simulink model "Counter_mod5"  (R2020a)
settings: Solver=VariableStepAuto  StartTime=0.0  StopTime=10  RelTol=1e-3
undefined symbols (not defined in the file): sigbuilder_block
settings Model: Creator=Shivam  LastModifiedBy=Shivam

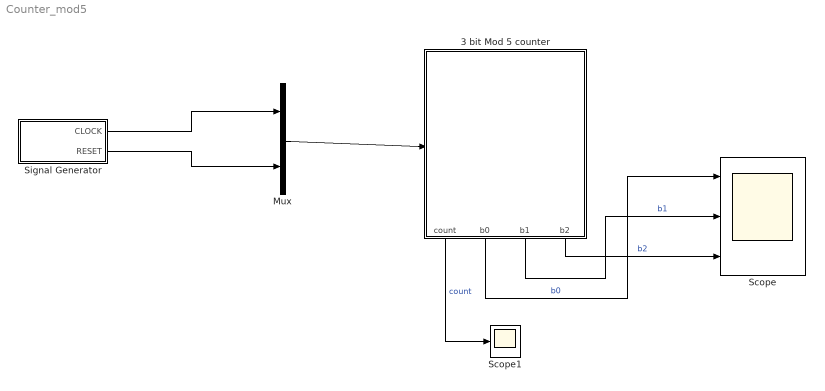
== system Counter_mod5 ==
  3 bit Mod 5 counter : Stateflow chart  TreatAsAtomicUnit=on
  Mux : Mux  Inputs=2
  Scope : Scope  NumInputPorts=3
  Scope1 : Scope
  Signal Generator : Subsystem  Tag=STV Subsys  LoadFcn=sigbuilder_block('load');  StartFcn=sigbuilder_block('start');  StopFcn=sigbuilder_block('stop');  ClipboardFcn=sigbuilder_block('clipboard');  mask(Sigbuilder block){tuvar=[0:10]}
      mask help: Simulink:masks:SigbuilderBlock_MD
      mask init:
      | if ~strcmp(get_param(bdroot(gcbh),'SimulationStatus'),'stopped') tuvar = sigbuilder_block('maskInit'); end
      settings: CopyFcn=sigbuilder_block('copy');  DeleteFcn=sigbuilder_block('delete');  ModelCloseFcn=sigbuilder_block('modelClose');  PreSaveFcn=sigbuilder_block('preSave');  PauseFcn=sigbuilder_block('pause');  ContinueFcn=sigbuilder_block('continue');  NameChangeFcn=sigbuilder_block('namechange');  OpenFcn=sigbuilder_block('open',[283.5 133.5 550.5 359.25 ]);  CloseFcn=sigbuilder_block('close');
      mask Display: plot(0, 0, 100, 100,[2, 2, 32, 32, 2], [68, 8, 8, 68, 68],[32, 2], [38, 38], [32, 19, 2],[53, 60, 44], [32, 17, 17, 2],[16, 16, 31, 31]);txt = getActiveGroup(gcbh);text(2, 100, txt,'verticalAlignment', 'top');
  wires:
  Mux/1 -> 3 bit Mod 5 counter/Trigger
  Signal Generator/1(CLOCK) -> Mux/1
  Signal Generator/2(RESET) -> Mux/2
  3 bit Mod 5 counter/2(b0) -> Scope/1  "b0"
  3 bit Mod 5 counter/3(b1) -> Scope/2  "b1"
  3 bit Mod 5 counter/4(b2) -> Scope/3  "b2"
  3 bit Mod 5 counter/1(count) -> Scope1/1  "count"

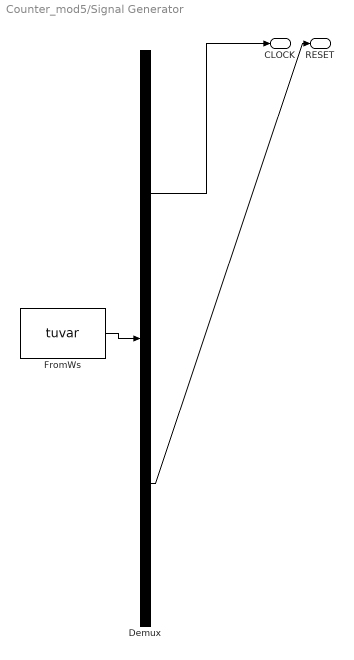
== system Counter_mod5/Signal Generator ==
  Demux : Demux  Tag=STV Demux  Outputs=2
      settings: DisplayOption=none
  FromWs : FromWorkspace  Tag=STV FromWs  VariableName=tuvar
      SigBuilderData=|
      | common.afterFinalStr = 'Extrapolate'
      | common.sampleTime = 0
      | dataSet.timeRange = [0 10]
      | dataSet.name = 'Group 1'
      | sbobj.Groups.Name = 'Group 1'
      | sbobj.Groups.Signals(1).Name = 'CLOCK'
      | sbobj.Groups.Signals(1).XData = [0 0.5 0.5 1 1 1.5 1.5 2 2 2.5 2.5 3 3 3.5 3.5 4 4 4.5 4.5 5 5 5.5 5.5 6 6 6.5 6.5 7 7 7.5 7.5 8 8 8.5 8.5 9 9 9.5 9.5 10]
      | sbobj.Groups.Signals(1).YData = [1 1 0 0 1 1 0 0 1 1 0 0 1 1 0 0 1 1 0 0 1 1 0 0 1 1 0 0 1 1 0 0 1 1 0 0 1 1 0 0]
      | sbobj.Groups.Signals(2).Name = 'RESET'
      | sbobj.Groups.Signals(2).XData = [0 7.98 7.98 9.02 9.02 10]
      | sbobj.Groups.Signals(2).YData = [0 0 1.02 1.02 0 0]
  CLOCK : Outport  Tag=STV Outport
  RESET : Outport  Tag=STV Outport  Port=2
  wires:
  FromWs/1 -> Demux/1
  Demux/1 -> CLOCK/1
  Demux/2 -> RESET/1

== stateflow chart Counter_mod5/3 bit Mod 5 counter ==
  settings: executeAtInitialization=1
  state State2
    entry:
    b0 =1;
    b1 = 0;
    b2 = 0;
    count = 1;
  state State3
    entry:
    b0 =0;
    b1 = 1;
    b2 = 0;
    count = 2;
  state State1
    entry:
    b0 =0;
    b1=0;
    b2=0;
    count =0;
  state State5
    entry:
    b0 =0;
    b1 = 0;
    b2 = 1;
    count = 4;
  state State4
    entry:
    b0 =1;
    b1 = 1;
    b2 = 0;
    count = 3;
  State2 -> State3 [order 2] : CLOCK
  State1 -> State2 : CLOCK
  (default) -> State1
  State2 -> State1 [order 1] : Reset
  State3 -> State1 [order 1] : Reset
  State3 -> State4 [order 2] : CLOCK
  State4 -> State1 [order 1] : Reset
  State5 -> State1 [order 1] : Reset
  State5 -> State1 [order 2] : CLOCK
  State4 -> State5 [order 2] : CLOCK
  data: count output; b0 output; b1 output; b2 output
  events: CLOCK input RISING_EDGE_EVENT; Reset input RISING_EDGE_EVENT
